simulink model "BasicRobot_RotationTest"  (R2023b)
settings: Solver=VariableStepAuto  StartTime=0.0  StopTime=10.0  RelTol=1e-3
values from neighbouring files (symbols this model uses):
  r = 0.15    [BasicRobot_Parameters.m]
settings Model: Creator=BeanieBabyJ  LastModifiedBy=BeanieBabyJ

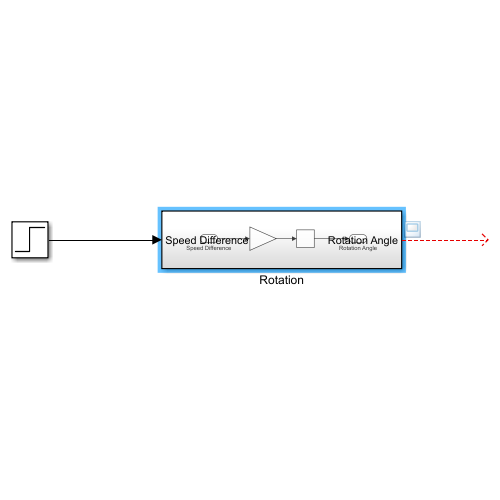
[thumbnail: Simulink's stored preview of the top-level diagram]
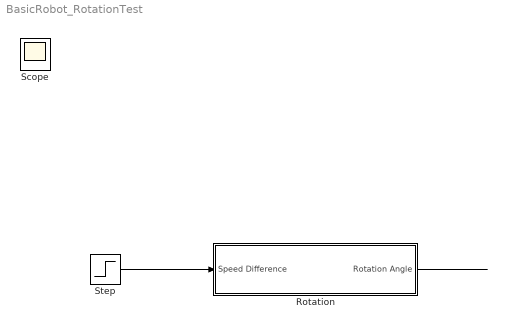
== system BasicRobot_RotationTest ==
  Rotation : Subsystem
  Step : Step  SampleTime=0
  Scope : Scope
  wires:
  Step/1 -> Rotation/1(Speed Difference)
  Rotation/1(Rotation Angle) -> ?

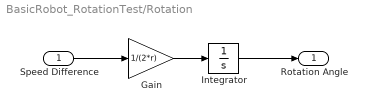
== system BasicRobot_RotationTest/Rotation ==
  Speed Difference : Inport
  Gain : Gain  Gain=1/(2*r)
  Integrator : Integrator
  Rotation Angle : Outport
  wires:
  Speed Difference/1 -> Gain/1
  Gain/1 -> Integrator/1
  Integrator/1 -> Rotation Angle/1
